simulink model "pipelined_simon"  (R2015b)
settings: Solver=FixedStepDiscrete  SolverMode=SingleTasking  StartTime=0.0  StopTime=5e-4  RelTol=1e-3
undefined symbols (not defined in the file or in its folder): a, b
libraries: shlslibv1 x1320
(part 1 of 6)
settings Model: synDspstartup=OK  Creator=pgali  LastModifiedBy=vchand32
settings DataIOCC: SaveOutput=off  SignalLogging=off  SaveTime=off
settings OptimizationCC: DefaultParameterBehavior=Inlined
settings DebuggingCC: AlgebraicLoopMsg=error  InheritedTsInSrcMsg=none

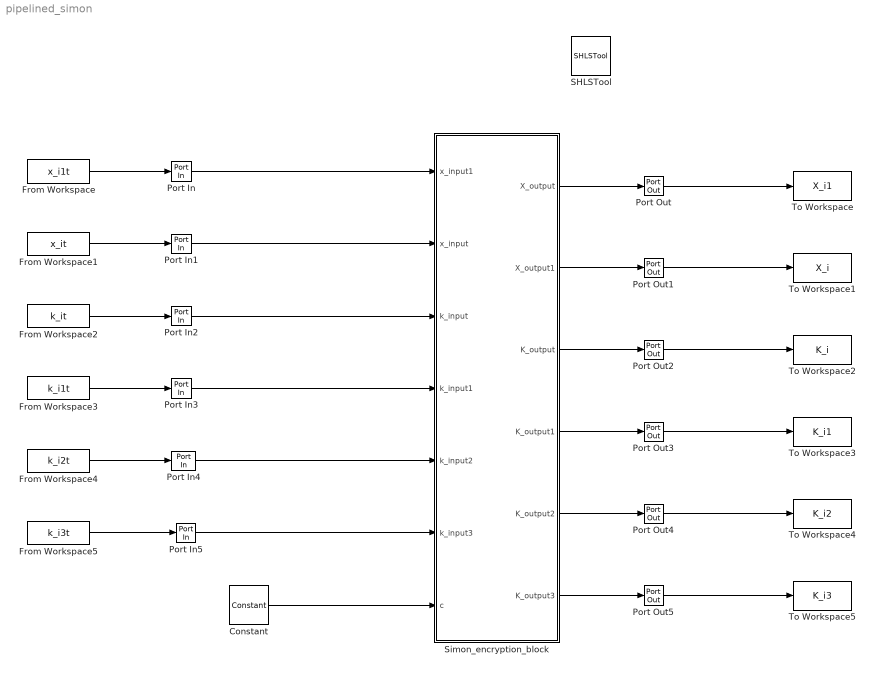
== system pipelined_simon ==
  Constant : shlslibv1/Sources/Constant  syn_cst_val=65532  syn_cst_format=Automatic  syn_cst_wl=1  syn_cst_fl=0  syn_cst_dt=unsigned  syn_cst_rnd=on  syn_cst_st=1/1040.5e6  synBlockType=primitive  synLatency=0  synBlockId=15
  From Workspace : FromWorkspace  VariableName=x_i1t  SampleTime=0
  From Workspace1 : FromWorkspace  VariableName=x_it  SampleTime=0
  From Workspace2 : FromWorkspace  VariableName=k_it  SampleTime=0
  From Workspace3 : FromWorkspace  VariableName=k_i1t  SampleTime=0
  From Workspace4 : FromWorkspace  VariableName=k_i2t  SampleTime=0
  From Workspace5 : FromWorkspace  VariableName=k_i3t  SampleTime=0
  Port In{,1..5} (6 alike) : shlslibv1/Ports & Subsystems/Port In  syn_out_wl=16  syn_out_fl=0  syn_out_dt=unsigned  syn_out_st=1/1040.5e6  syn_capture=on  syn_register=on  syn_out_sat=off  syn_out_rnd=on  synBlockType=port  synLatency=1  synBlockId=0
  Port Out{,1..5} (6 alike) : shlslibv1/Ports & Subsystems/Port Out  syn_capture=on  syn_register=on  synBlockType=port  synLatency=1  synBlockId=1
  SHLSTool : shlslibv1/SHLSTool  synBlockType=tool  syn_dsp_mode=FPGA
  "Simon_encryption_block " : Subsystem
  To Workspace : ToWorkspace  VariableName=X_i1  SaveFormat=Structure With Time  SampleTime=-1
  To Workspace1 : ToWorkspace  VariableName=X_i  SaveFormat=Structure With Time  SampleTime=-1
  To Workspace2 : ToWorkspace  VariableName=K_i  SaveFormat=Structure With Time  SampleTime=-1
  To Workspace3 : ToWorkspace  VariableName=K_i1  SaveFormat=Structure With Time  SampleTime=-1
  To Workspace4 : ToWorkspace  VariableName=K_i2  SaveFormat=Structure With Time  SampleTime=-1
  To Workspace5 : ToWorkspace  VariableName=K_i3  SaveFormat=Structure With Time  SampleTime=-1
  wires:
  From Workspace1/1 -> Port In1/1
  From Workspace2/1 -> Port In2/1
  From Workspace/1 -> Port In/1
  From Workspace3/1 -> Port In3/1
  From Workspace4/1 -> Port In4/1
  From Workspace5/1 -> Port In5/1
  Port In/1 -> "Simon_encryption_block "/1(x_input1)
  Port In1/1 -> "Simon_encryption_block "/2(x_input)
  Port In2/1 -> "Simon_encryption_block "/3(k_input)
  Port In3/1 -> "Simon_encryption_block "/4(k_input1)
  Port In4/1 -> "Simon_encryption_block "/5(k_input2)
  Port In5/1 -> "Simon_encryption_block "/6(k_input3)
  Port Out/1 -> To Workspace/1
  Port Out1/1 -> To Workspace1/1
  Port Out3/1 -> To Workspace3/1
  Port Out4/1 -> To Workspace4/1
  Port Out5/1 -> To Workspace5/1
  Port Out2/1 -> To Workspace2/1
  "Simon_encryption_block "/1(X_output) -> Port Out/1
  "Simon_encryption_block "/2(X_output1) -> Port Out1/1
  "Simon_encryption_block "/3(K_output) -> Port Out2/1
  "Simon_encryption_block "/4(K_output1) -> Port Out3/1
  "Simon_encryption_block "/5(K_output2) -> Port Out4/1
  "Simon_encryption_block "/6(K_output3) -> Port Out5/1
  Constant/1 -> "Simon_encryption_block "/7(c)

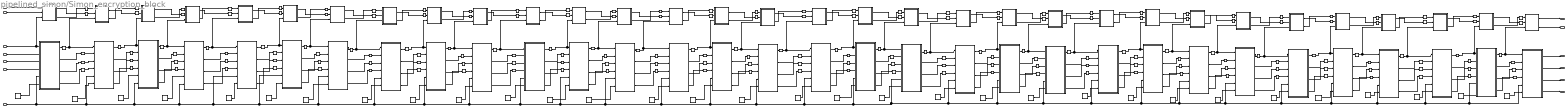
== system pipelined_simon/Simon_encryption_block  ==
  x_input1 : Inport
  x_input : Inport  Port=2
  k_input : Inport  Port=3
  k_input1 : Inport  Port=4
  k_input2 : Inport  Port=5
  k_input3 : Inport  Port=6
  c : Inport  Port=7
  Delay{1..186} (186 alike) : shlslibv1/Memories/Delay  syn_delay_val=1  synBlockType=primitive  synLatency=1  synBlockId=104
  Key_expansion_block : Subsystem
  Key_expansion_block1 : Subsystem
  Key_expansion_block10 : Subsystem
  Key_expansion_block11 : Subsystem
  Key_expansion_block12 : Subsystem
  Key_expansion_block13 : Subsystem
  Key_expansion_block14 : Subsystem
  Key_expansion_block15 : Subsystem
  Key_expansion_block16 : Subsystem
  Key_expansion_block17 : Subsystem
  Key_expansion_block18 : Subsystem
  Key_expansion_block19 : Subsystem
  Key_expansion_block2 : Subsystem
  Key_expansion_block20 : Subsystem
  Key_expansion_block21 : Subsystem
  Key_expansion_block22 : Subsystem
  Key_expansion_block23 : Subsystem
  Key_expansion_block24 : Subsystem
  Key_expansion_block25 : Subsystem
  Key_expansion_block26 : Subsystem
  Key_expansion_block27 : Subsystem
  Key_expansion_block28 : Subsystem
  Key_expansion_block29 : Subsystem
  Key_expansion_block3 : Subsystem
  Key_expansion_block30 : Subsystem
  Key_expansion_block31 : Subsystem
  Key_expansion_block4 : Subsystem
  Key_expansion_block5 : Subsystem
  Key_expansion_block6 : Subsystem
  Key_expansion_block7 : Subsystem
  Key_expansion_block8 : Subsystem
  Key_expansion_block9 : Subsystem
  Round_block : Subsystem
  Round_block1 : Subsystem
  Round_block10 : Subsystem
  Round_block11 : Subsystem
  Round_block12 : Subsystem
  Round_block13 : Subsystem
  Round_block14 : Subsystem
  Round_block15 : Subsystem
  Round_block16 : Subsystem
  Round_block17 : Subsystem
  Round_block18 : Subsystem
  Round_block19 : Subsystem
  Round_block2 : Subsystem
  Round_block20 : Subsystem
  Round_block21 : Subsystem
  Round_block22 : Subsystem
  Round_block23 : Subsystem
  Round_block24 : Subsystem
  Round_block25 : Subsystem
  Round_block26 : Subsystem
  Round_block27 : Subsystem
  Round_block28 : Subsystem
  Round_block29 : Subsystem
  Round_block3 : Subsystem
  Round_block30 : Subsystem
  Round_block31 : Subsystem
  Round_block4 : Subsystem
  Round_block5 : Subsystem
  Round_block6 : Subsystem
  Round_block7 : Subsystem
  Round_block8 : Subsystem
  Round_block9 : Subsystem
  Sequence{,1..4,6,10,13,15,17..18,23..25,28..29} (16 alike) : shlslibv1/Sources/Sequence  syn_seq_vec=[1]  syn_seq_wl=16  syn_seq_fl=0  syn_seq_dt=unsigned  syn_rst_port=off  syn_en_port=off  syn_seq_st=-1  synBlockType=custom  synLatency=1
  Sequence{5,7..9,11..12,14,16,19..22,26..27,30..31} (16 alike) : shlslibv1/Sources/Sequence  syn_seq_vec=[0]  syn_seq_wl=16  syn_seq_fl=0  syn_seq_dt=unsigned  syn_rst_port=off  syn_en_port=off  syn_seq_st=-1  synBlockType=custom  synLatency=1
  X_output : Outport
  X_output1 : Outport  Port=2
  K_output : Outport  Port=3
  K_output1 : Outport  Port=4
  K_output2 : Outport  Port=5
  K_output3 : Outport  Port=6
  wires:
  Key_expansion_block/2(Key_output1) -> Delay11/1
  Key_expansion_block/3(Key_output2) -> Delay12/1
  Key_expansion_block/4(Key_output3) -> Delay13/1
  x_input1/1 -> Round_block/1(" x_input1")
  x_input/1 -> Round_block/2(x_input)
  k_input/1 -> Round_block/3(k_i), Key_expansion_block/1(key_input)
  k_input1/1 -> Key_expansion_block/2(key_input1)
  k_input2/1 -> Key_expansion_block/3(key_input2)
  k_input3/1 -> Key_expansion_block/4(key_input3)
  Round_block/2(X_output) -> Delay7/1
  Round_block/1(X_output1) -> Delay8/1
  Round_block1/1(X_output1) -> Delay15/1
  Round_block1/2(X_output) -> Delay14/1
  Key_expansion_block1/2(Key_output1) -> Delay18/1
  Key_expansion_block1/3(Key_output2) -> Delay19/1
  Key_expansion_block1/4(Key_output3) -> Delay20/1
  Round_block2/1(X_output1) -> Delay22/1
  Round_block2/2(X_output) -> Delay21/1
  Key_expansion_block2/2(Key_output1) -> Delay25/1
  Key_expansion_block2/3(Key_output2) -> Delay26/1
  Key_expansion_block2/4(Key_output3) -> Delay27/1
  Delay7/1 -> Round_block1/1(" x_input1")
  Delay8/1 -> Round_block1/2(x_input)
  Key_expansion_block/1(Key_output) -> Delay9/1
  Delay11/1 -> Key_expansion_block1/2(key_input1)
  Delay12/1 -> Key_expansion_block1/3(key_input2)
  Delay13/1 -> Key_expansion_block1/4(key_input3)
  Delay14/1 -> Round_block2/1(" x_input1")
  Delay15/1 -> Round_block2/2(x_input)
  Key_expansion_block1/1(Key_output) -> Delay10/1
  Delay18/1 -> Key_expansion_block2/2(key_input1)
  Delay19/1 -> Key_expansion_block2/3(key_input2)
  Delay20/1 -> Key_expansion_block2/4(key_input3)
  Delay21/1 -> Round_block3/1(" x_input1")
  Delay22/1 -> Round_block3/2(x_input)
  Key_expansion_block2/1(Key_output) -> Delay16/1
  Delay25/1 -> Key_expansion_block3/2(key_input1)
  Delay26/1 -> Key_expansion_block3/3(key_input2)
  Delay27/1 -> Key_expansion_block3/4(key_input3)
  Delay9/1 -> Round_block1/3(k_i), Key_expansion_block1/1(key_input)
  Delay10/1 -> Round_block2/3(k_i), Key_expansion_block2/1(key_input)
  Delay16/1 -> Round_block3/3(k_i), Key_expansion_block3/1(key_input)
  Key_expansion_block3/2(Key_output1) -> Delay2/1
  Key_expansion_block3/3(Key_output2) -> Delay3/1
  Key_expansion_block3/4(Key_output3) -> Delay4/1
  Round_block3/2(X_output) -> Delay34/1
  Round_block3/1(X_output1) -> Delay35/1
  Round_block4/1(X_output1) -> Delay6/1
  Round_block4/2(X_output) -> Delay5/1
  Key_expansion_block4/2(Key_output1) -> Delay23/1
  Key_expansion_block4/3(Key_output2) -> Delay24/1
  Key_expansion_block4/4(Key_output3) -> Delay28/1
  Round_block5/1(X_output1) -> Delay30/1
  Round_block5/2(X_output) -> Delay29/1
  Key_expansion_block5/2(Key_output1) -> Delay31/1
  Key_expansion_block5/3(Key_output2) -> Delay32/1
  Key_expansion_block5/4(Key_output3) -> Delay33/1
  Delay34/1 -> Round_block4/1(" x_input1")
  Delay35/1 -> Round_block4/2(x_input)
  Key_expansion_block3/1(Key_output) -> Delay36/1
  Delay2/1 -> Key_expansion_block4/2(key_input1)
  Delay3/1 -> Key_expansion_block4/3(key_input2)
  Delay4/1 -> Key_expansion_block4/4(key_input3)
  Delay5/1 -> Round_block5/1(" x_input1")
  Delay6/1 -> Round_block5/2(x_input)
  Key_expansion_block4/1(Key_output) -> Delay1/1
  Delay23/1 -> Key_expansion_block5/2(key_input1)
  Delay24/1 -> Key_expansion_block5/3(key_input2)
  Delay28/1 -> Key_expansion_block5/4(key_input3)
  Delay29/1 -> Round_block6/1(" x_input1")
  Delay30/1 -> Round_block6/2(x_input)
  Key_expansion_block5/1(Key_output) -> Delay17/1
  Delay31/1 -> Key_expansion_block6/2(key_input1)
  Delay32/1 -> Key_expansion_block6/3(key_input2)
  Delay33/1 -> Key_expansion_block6/4(key_input3)
  Delay36/1 -> Round_block4/3(k_i), Key_expansion_block4/1(key_input)
  Delay1/1 -> Round_block5/3(k_i), Key_expansion_block5/1(key_input)
  Delay17/1 -> Round_block6/3(k_i), Key_expansion_block6/1(key_input)
  Key_expansion_block6/2(Key_output1) -> Delay39/1
  Key_expansion_block6/3(Key_output2) -> Delay40/1
  Key_expansion_block6/4(Key_output3) -> Delay41/1
  Round_block6/2(X_output) -> Delay70/1
  Round_block6/1(X_output1) -> Delay71/1
  Round_block7/1(X_output1) -> Delay43/1
  Round_block7/2(X_output) -> Delay42/1
  Key_expansion_block7/2(Key_output1) -> Delay46/1
  Key_expansion_block7/3(Key_output2) -> Delay47/1
  Key_expansion_block7/4(Key_output3) -> Delay49/1
  Round_block8/1(X_output1) -> Delay51/1
  Round_block8/2(X_output) -> Delay50/1
  Key_expansion_block8/2(Key_output1) -> Delay54/1
  Key_expansion_block8/3(Key_output2) -> Delay55/1
  Key_expansion_block8/4(Key_output3) -> Delay56/1
  Delay70/1 -> Round_block7/1(" x_input1")
  Delay71/1 -> Round_block7/2(x_input)
  Key_expansion_block6/1(Key_output) -> Delay72/1
  Delay39/1 -> Key_expansion_block7/2(key_input1)
  Delay40/1 -> Key_expansion_block7/3(key_input2)
  Delay41/1 -> Key_expansion_block7/4(key_input3)
  Delay42/1 -> Round_block8/1(" x_input1")
  Delay43/1 -> Round_block8/2(x_input)
  Key_expansion_block7/1(Key_output) -> Delay38/1
  Delay46/1 -> Key_expansion_block8/2(key_input1)
  Delay47/1 -> Key_expansion_block8/3(key_input2)
  Delay49/1 -> Key_expansion_block8/4(key_input3)
  Delay50/1 -> Round_block9/1(" x_input1")
  Delay51/1 -> Round_block9/2(x_input)
  Key_expansion_block8/1(Key_output) -> Delay44/1
  Delay54/1 -> Key_expansion_block9/2(key_input1)
  Delay55/1 -> Key_expansion_block9/3(key_input2)
  Delay56/1 -> Key_expansion_block9/4(key_input3)
  Delay72/1 -> Round_block7/3(k_i), Key_expansion_block7/1(key_input)
  Delay38/1 -> Round_block8/3(k_i), Key_expansion_block8/1(key_input)
  Delay44/1 -> Round_block9/3(k_i), Key_expansion_block9/1(key_input)
  Key_expansion_block9/2(Key_output1) -> Delay48/1
  Key_expansion_block9/3(Key_output2) -> Delay59/1
  Key_expansion_block9/4(Key_output3) -> Delay67/1
  Round_block9/2(X_output) -> Delay64/1
  Round_block9/1(X_output1) -> Delay65/1
  Round_block10/1(X_output1) -> Delay69/1
  Round_block10/2(X_output) -> Delay68/1
  Key_expansion_block10/2(Key_output1) -> Delay52/1
  Key_expansion_block10/3(Key_output2) -> Delay53/1
  Key_expansion_block10/4(Key_output3) -> Delay57/1
  Round_block11/1(X_output1) -> Delay60/1
  Round_block11/2(X_output) -> Delay58/1
  Key_expansion_block11/2(Key_output1) -> Delay61/1
  Key_expansion_block11/3(Key_output2) -> Delay62/1
  Key_expansion_block11/4(Key_output3) -> Delay63/1
  Delay64/1 -> Round_block10/1(" x_input1")
  Delay65/1 -> Round_block10/2(x_input)
  Key_expansion_block9/1(Key_output) -> Delay66/1
  Delay48/1 -> Key_expansion_block10/2(key_input1)
  Delay59/1 -> Key_expansion_block10/3(key_input2)
  Delay67/1 -> Key_expansion_block10/4(key_input3)
  Delay68/1 -> Round_block11/1(" x_input1")
  Delay69/1 -> Round_block11/2(x_input)
  Key_expansion_block10/1(Key_output) -> Delay37/1
  Delay52/1 -> Key_expansion_block11/2(key_input1)
  Delay53/1 -> Key_expansion_block11/3(key_input2)
  Delay57/1 -> Key_expansion_block11/4(key_input3)
  Delay58/1 -> Round_block12/1(" x_input1")
  Delay60/1 -> Round_block12/2(x_input)
  Key_expansion_block11/1(Key_output) -> Delay45/1
  Delay61/1 -> Key_expansion_block12/2(key_input1)
  Delay62/1 -> Key_expansion_block12/3(key_input2)
  Delay63/1 -> Key_expansion_block12/4(key_input3)
  Delay66/1 -> Round_block10/3(k_i), Key_expansion_block10/1(key_input)
  Delay37/1 -> Round_block11/3(k_i), Key_expansion_block11/1(key_input)
  Delay45/1 -> Round_block12/3(k_i), Key_expansion_block12/1(key_input)
  Key_expansion_block12/2(Key_output1) -> Delay75/1
  Key_expansion_block12/3(Key_output2) -> Delay76/1
  Key_expansion_block12/4(Key_output3) -> Delay77/1
  Round_block12/2(X_output) -> Delay139/1
  Round_block12/1(X_output1) -> Delay143/1
  Round_block13/1(X_output1) -> Delay79/1
  Round_block13/2(X_output) -> Delay78/1
  Key_expansion_block13/2(Key_output1) -> Delay82/1
  Key_expansion_block13/3(Key_output2) -> Delay83/1
  Key_expansion_block13/4(Key_output3) -> Delay85/1
  Round_block14/1(X_output1) -> Delay87/1
  Round_block14/2(X_output) -> Delay86/1
  Key_expansion_block14/2(Key_output1) -> Delay90/1
  Key_expansion_block14/3(Key_output2) -> Delay91/1
  Key_expansion_block14/4(Key_output3) -> Delay92/1
  Delay139/1 -> Round_block13/1(" x_input1")
  Delay143/1 -> Round_block13/2(x_input)
  Key_expansion_block12/1(Key_output) -> Delay144/1
  Delay75/1 -> Key_expansion_block13/2(key_input1)
  Delay76/1 -> Key_expansion_block13/3(key_input2)
  Delay77/1 -> Key_expansion_block13/4(key_input3)
  Delay78/1 -> Round_block14/1(" x_input1")
  Delay79/1 -> Round_block14/2(x_input)
  Key_expansion_block13/1(Key_output) -> Delay74/1
  Delay82/1 -> Key_expansion_block14/2(key_input1)
  Delay83/1 -> Key_expansion_block14/3(key_input2)
  Delay85/1 -> Key_expansion_block14/4(key_input3)
  Delay86/1 -> Round_block15/1(" x_input1")
  Delay87/1 -> Round_block15/2(x_input)
  Key_expansion_block14/1(Key_output) -> Delay80/1
  Delay90/1 -> Key_expansion_block15/2(key_input1)
  Delay91/1 -> Key_expansion_block15/3(key_input2)
  Delay92/1 -> Key_expansion_block15/4(key_input3)
  Delay144/1 -> Round_block13/3(k_i), Key_expansion_block13/1(key_input)
  Delay74/1 -> Round_block14/3(k_i), Key_expansion_block14/1(key_input)
  Delay80/1 -> Round_block15/3(k_i), Key_expansion_block15/1(key_input)
  Key_expansion_block15/2(Key_output1) -> Delay84/1
  Key_expansion_block15/3(Key_output2) -> Delay95/1
  Key_expansion_block15/4(Key_output3) -> Delay106/1
  Round_block15/2(X_output) -> Delay100/1
  Round_block15/1(X_output1) -> Delay101/1
  Round_block16/1(X_output1) -> Delay128/1
  Round_block16/2(X_output) -> Delay117/1
  Key_expansion_block16/2(Key_output1) -> Delay88/1
  Key_expansion_block16/3(Key_output2) -> Delay89/1
  Key_expansion_block16/4(Key_output3) -> Delay93/1
  Round_block17/1(X_output1) -> Delay96/1
  Round_block17/2(X_output) -> Delay94/1
  Key_expansion_block17/2(Key_output1) -> Delay97/1
  Key_expansion_block17/3(Key_output2) -> Delay98/1
  Key_expansion_block17/4(Key_output3) -> Delay99/1
  Delay100/1 -> Round_block16/1(" x_input1")
  Delay101/1 -> Round_block16/2(x_input)
  Key_expansion_block15/1(Key_output) -> Delay102/1
  Delay84/1 -> Key_expansion_block16/2(key_input1)
  Delay95/1 -> Key_expansion_block16/3(key_input2)
  Delay106/1 -> Key_expansion_block16/4(key_input3)
  Delay117/1 -> Round_block17/1(" x_input1")
  Delay128/1 -> Round_block17/2(x_input)
  Key_expansion_block16/1(Key_output) -> Delay73/1
  Delay88/1 -> Key_expansion_block17/2(key_input1)
  Delay89/1 -> Key_expansion_block17/3(key_input2)
  Delay93/1 -> Key_expansion_block17/4(key_input3)
  Delay94/1 -> Round_block18/1(" x_input1")
  Delay96/1 -> Round_block18/2(x_input)
  Key_expansion_block17/1(Key_output) -> Delay81/1
  Delay97/1 -> Key_expansion_block18/2(key_input1)
  Delay98/1 -> Key_expansion_block18/3(key_input2)
  Delay99/1 -> Key_expansion_block18/4(key_input3)
  Delay102/1 -> Round_block16/3(k_i), Key_expansion_block16/1(key_input)
  Delay73/1 -> Round_block17/3(k_i), Key_expansion_block17/1(key_input)
  Delay81/1 -> Round_block18/3(k_i), Key_expansion_block18/1(key_input)
  Key_expansion_block18/2(Key_output1) -> Delay105/1
  Key_expansion_block18/3(Key_output2) -> Delay107/1
  Key_expansion_block18/4(Key_output3) -> Delay108/1
  Round_block18/2(X_output) -> Delay140/1
  Round_block18/1(X_output1) -> Delay141/1
  Round_block19/1(X_output1) -> Delay110/1
  Round_block19/2(X_output) -> Delay109/1
  Key_expansion_block19/2(Key_output1) -> Delay113/1
  Key_expansion_block19/3(Key_output2) -> Delay114/1
  Key_expansion_block19/4(Key_output3) -> Delay116/1
  Round_block20/1(X_output1) -> Delay119/1
  Round_block20/2(X_output) -> Delay118/1
  Key_expansion_block20/2(Key_output1) -> Delay122/1
  Key_expansion_block20/3(Key_output2) -> Delay123/1
  Key_expansion_block20/4(Key_output3) -> Delay124/1
  Delay140/1 -> Round_block19/1(" x_input1")
  Delay141/1 -> Round_block19/2(x_input)
  Key_expansion_block18/1(Key_output) -> Delay142/1
  Delay105/1 -> Key_expansion_block19/2(key_input1)
  Delay107/1 -> Key_expansion_block19/3(key_input2)
  Delay108/1 -> Key_expansion_block19/4(key_input3)
  Delay109/1 -> Round_block20/1(" x_input1")
  Delay110/1 -> Round_block20/2(x_input)
  Key_expansion_block19/1(Key_output) -> Delay104/1
  Delay113/1 -> Key_expansion_block20/2(key_input1)
  Delay114/1 -> Key_expansion_block20/3(key_input2)
  Delay116/1 -> Key_expansion_block20/4(key_input3)
  Delay118/1 -> Round_block21/1(" x_input1")
  Delay119/1 -> Round_block21/2(x_input)
  Key_expansion_block20/1(Key_output) -> Delay111/1
  Delay122/1 -> Key_expansion_block21/2(key_input1)
  Delay123/1 -> Key_expansion_block21/3(key_input2)
  Delay124/1 -> Key_expansion_block21/4(key_input3)
  Delay142/1 -> Round_block19/3(k_i), Key_expansion_block19/1(key_input)
  Delay104/1 -> Round_block20/3(k_i), Key_expansion_block20/1(key_input)
  Delay111/1 -> Round_block21/3(k_i), Key_expansion_block21/1(key_input)
  Key_expansion_block21/2(Key_output1) -> Delay115/1
  Key_expansion_block21/3(Key_output2) -> Delay127/1
  Key_expansion_block21/4(Key_output3) -> Delay136/1
  Round_block21/2(X_output) -> Delay133/1
  Round_block21/1(X_output1) -> Delay134/1
  Round_block22/1(X_output1) -> Delay138/1
  Round_block22/2(X_output) -> Delay137/1
  Key_expansion_block22/2(Key_output1) -> Delay120/1
  Key_expansion_block22/3(Key_output2) -> Delay121/1
  Key_expansion_block22/4(Key_output3) -> Delay125/1
  Round_block23/1(X_output1) -> Delay129/1
  Round_block23/2(X_output) -> Delay126/1
  Key_expansion_block23/2(Key_output1) -> Delay130/1
  Key_expansion_block23/3(Key_output2) -> Delay131/1
  Key_expansion_block23/4(Key_output3) -> Delay132/1
  Delay133/1 -> Round_block22/1(" x_input1")
  Delay134/1 -> Round_block22/2(x_input)
  Key_expansion_block21/1(Key_output) -> Delay135/1
  Delay115/1 -> Key_expansion_block22/2(key_input1)
  Delay127/1 -> Key_expansion_block22/3(key_input2)
  Delay136/1 -> Key_expansion_block22/4(key_input3)
  Delay137/1 -> Round_block23/1(" x_input1")
  Delay138/1 -> Round_block23/2(x_input)
  Key_expansion_block22/1(Key_output) -> Delay103/1
  Delay120/1 -> Key_expansion_block23/2(key_input1)
  Delay121/1 -> Key_expansion_block23/3(key_input2)
  Delay125/1 -> Key_expansion_block23/4(key_input3)
  Delay126/1 -> Round_block24/1(" x_input1")
  Delay129/1 -> Round_block24/2(x_input)
  Key_expansion_block23/1(Key_output) -> Delay112/1
  Delay130/1 -> Key_expansion_block24/2(key_input1)
  Delay131/1 -> Key_expansion_block24/3(key_input2)
  Delay132/1 -> Key_expansion_block24/4(key_input3)
  Delay135/1 -> Round_block22/3(k_i), Key_expansion_block22/1(key_input)
  Delay103/1 -> Round_block23/3(k_i), Key_expansion_block23/1(key_input)
  Delay112/1 -> Round_block24/3(k_i), Key_expansion_block24/1(key_input)
  Round_block24/1(X_output1) -> Delay183/1
  Round_block24/2(X_output) -> Delay182/1
  Key_expansion_block24/2(Key_output1) -> Delay184/1
  Key_expansion_block24/3(Key_output2) -> Delay185/1
  Key_expansion_block24/4(Key_output3) -> Delay186/1
  Delay182/1 -> Round_block25/1(" x_input1")
  Delay183/1 -> Round_block25/2(x_input)
  Key_expansion_block24/1(Key_output) -> Delay181/1
  Delay184/1 -> Key_expansion_block25/2(key_input1)
  Delay185/1 -> Key_expansion_block25/3(key_input2)
  Delay186/1 -> Key_expansion_block25/4(key_input3)
  Delay181/1 -> Round_block25/3(k_i), Key_expansion_block25/1(key_input)
  Key_expansion_block25/2(Key_output1) -> Delay147/1
  Key_expansion_block25/3(Key_output2) -> Delay148/1
  Key_expansion_block25/4(Key_output3) -> Delay149/1
  Sequence27/1 -> Key_expansion_block27/6(z)
  Sequence28/1 -> Key_expansion_block28/6(z)
  Round_block25/2(X_output) -> Delay178/1
  Round_block25/1(X_output1) -> Delay179/1
  Round_block26/1(X_output1) -> Delay151/1
  Round_block26/2(X_output) -> Delay150/1
  Key_expansion_block26/2(Key_output1) -> Delay154/1
  Key_expansion_block26/3(Key_output2) -> Delay155/1
  Key_expansion_block26/4(Key_output3) -> Delay157/1
  Round_block27/1(X_output1) -> Delay159/1
  Round_block27/2(X_output) -> Delay158/1
  Key_expansion_block27/2(Key_output1) -> Delay162/1
  Key_expansion_block27/3(Key_output2) -> Delay163/1
  Key_expansion_block27/4(Key_output3) -> Delay164/1
  Delay178/1 -> Round_block26/1(" x_input1")
  Delay179/1 -> Round_block26/2(x_input)
  Key_expansion_block25/1(Key_output) -> Delay180/1
  Delay147/1 -> Key_expansion_block26/2(key_input1)
  Delay148/1 -> Key_expansion_block26/3(key_input2)
  Delay149/1 -> Key_expansion_block26/4(key_input3)
  Delay150/1 -> Round_block27/1(" x_input1")
  Delay151/1 -> Round_block27/2(x_input)
  Key_expansion_block26/1(Key_output) -> Delay146/1
  Delay154/1 -> Key_expansion_block27/2(key_input1)
  Delay155/1 -> Key_expansion_block27/3(key_input2)
  Delay157/1 -> Key_expansion_block27/4(key_input3)
  Delay158/1 -> Round_block28/1(" x_input1")
  Delay159/1 -> Round_block28/2(x_input)
  Key_expansion_block27/1(Key_output) -> Delay152/1
  Delay162/1 -> Key_expansion_block28/2(key_input1)
  Delay163/1 -> Key_expansion_block28/3(key_input2)
  Delay164/1 -> Key_expansion_block28/4(key_input3)
  Delay180/1 -> Round_block26/3(k_i), Key_expansion_block26/1(key_input)
  Delay146/1 -> Round_block27/3(k_i), Key_expansion_block27/1(key_input)
  Delay152/1 -> Round_block28/3(k_i), Key_expansion_block28/1(key_input)
  Key_expansion_block28/2(Key_output1) -> Delay156/1
  Key_expansion_block28/3(Key_output2) -> Delay167/1
  Key_expansion_block28/4(Key_output3) -> Delay175/1
  Sequence30/1 -> Key_expansion_block30/6(z)
  Round_block28/2(X_output) -> Delay172/1
  Round_block28/1(X_output1) -> Delay173/1
  Round_block29/1(X_output1) -> Delay177/1
  Round_block29/2(X_output) -> Delay176/1
  Key_expansion_block29/2(Key_output1) -> Delay160/1
  Key_expansion_block29/3(Key_output2) -> Delay161/1
  Key_expansion_block29/4(Key_output3) -> Delay165/1
  Round_block30/1(X_output1) -> Delay168/1
  Round_block30/2(X_output) -> Delay166/1
  Key_expansion_block30/2(Key_output1) -> Delay169/1
  Key_expansion_block30/3(Key_output2) -> Delay170/1
  Key_expansion_block30/4(Key_output3) -> Delay171/1
  Delay172/1 -> Round_block29/1(" x_input1")
  Delay173/1 -> Round_block29/2(x_input)
  Key_expansion_block28/1(Key_output) -> Delay174/1
  Delay156/1 -> Key_expansion_block29/2(key_input1)
  Delay167/1 -> Key_expansion_block29/3(key_input2)
  Delay175/1 -> Key_expansion_block29/4(key_input3)
  Delay176/1 -> Round_block30/1(" x_input1")
  Delay177/1 -> Round_block30/2(x_input)
  Key_expansion_block29/1(Key_output) -> Delay145/1
  Delay160/1 -> Key_expansion_block30/2(key_input1)
  Delay161/1 -> Key_expansion_block30/3(key_input2)
  Delay165/1 -> Key_expansion_block30/4(key_input3)
  Delay166/1 -> Round_block31/1(" x_input1")
  Delay168/1 -> Round_block31/2(x_input)
  Key_expansion_block30/1(Key_output) -> Delay153/1
  Delay169/1 -> Key_expansion_block31/2(key_input1)
  Delay170/1 -> Key_expansion_block31/3(key_input2)
  Delay171/1 -> Key_expansion_block31/4(key_input3)
  Delay174/1 -> Round_block29/3(k_i), Key_expansion_block29/1(key_input)
  Delay145/1 -> Round_block30/3(k_i), Key_expansion_block30/1(key_input)
  Delay153/1 -> Round_block31/3(k_i), Key_expansion_block31/1(key_input)
  c/1 -> Key_expansion_block1/5(c), Key_expansion_block2/6(z), Key_expansion_block3/6(z), Key_expansion_block4/5(c), Key_expansion_block5/5(c), Key_expansion_block6/5(c), Key_expansion_block7/5(c), Key_expansion_block8/5(c), Key_expansion_block9/5(c), Key_expansion_block10/5(c), Key_expansion_block11/5(c), Key_expansion_block12/5(c), Key_expansion_block13/5(c), Key_expansion_block14/5(c), Key_expansion_block15/5(c), Key_expansion_block16/5(c), Key_expansion_block17/5(c), Key_expansion_block18/5(c), Key_expansion_block19/5(c), Key_expansion_block20/5(c), Key_expansion_block21/5(c), Key_expansion_block22/5(c), Key_expansion_block23/5(c), Key_expansion_block24/5(c), Key_expansion_block25/5(c), Key_expansion_block26/5(c), Key_expansion_block27/5(c), Key_expansion_block28/5(c), Key_expansion_block29/5(c), Key_expansion_block30/5(c), Key_expansion_block31/5(c), Key_expansion_block/5(c)
  Sequence/1 -> Key_expansion_block/6(z)
  Sequence1/1 -> Key_expansion_block1/6(z)
  Sequence2/1 -> Key_expansion_block2/5(c)
  Sequence3/1 -> Key_expansion_block3/5(c)
  Sequence4/1 -> Key_expansion_block4/6(z)
  Sequence5/1 -> Key_expansion_block5/6(z)
  Sequence6/1 -> Key_expansion_block6/6(z)
  Sequence7/1 -> Key_expansion_block7/6(z)
  Sequence8/1 -> Key_expansion_block8/6(z)
  Sequence9/1 -> Key_expansion_block9/6(z)
  Sequence10/1 -> Key_expansion_block10/6(z)
  Sequence11/1 -> Key_expansion_block11/6(z)
  Sequence12/1 -> Key_expansion_block12/6(z)
  Sequence13/1 -> Key_expansion_block13/6(z)
  Sequence14/1 -> Key_expansion_block14/6(z)
  Sequence15/1 -> Key_expansion_block15/6(z)
  Sequence16/1 -> Key_expansion_block16/6(z)
  Sequence17/1 -> Key_expansion_block17/6(z)
  Sequence18/1 -> Key_expansion_block18/6(z)
  Sequence19/1 -> Key_expansion_block19/6(z)
  Sequence20/1 -> Key_expansion_block20/6(z)
  Sequence21/1 -> Key_expansion_block21/6(z)
  Sequence22/1 -> Key_expansion_block22/6(z)
  Sequence23/1 -> Key_expansion_block23/6(z)
  Sequence29/1 -> Key_expansion_block29/6(z)
  Sequence26/1 -> Key_expansion_block26/6(z)
  Sequence31/1 -> Key_expansion_block31/6(z)
  Sequence25/1 -> Key_expansion_block25/6(z)
  Sequence24/1 -> Key_expansion_block24/6(z)
  Round_block31/1(X_output1) -> X_output/1
  Round_block31/2(X_output) -> X_output1/1
  Key_expansion_block31/1(Key_output) -> K_output/1
  Key_expansion_block31/2(Key_output1) -> K_output1/1
  Key_expansion_block31/3(Key_output2) -> K_output2/1
  Key_expansion_block31/4(Key_output3) -> K_output3/1

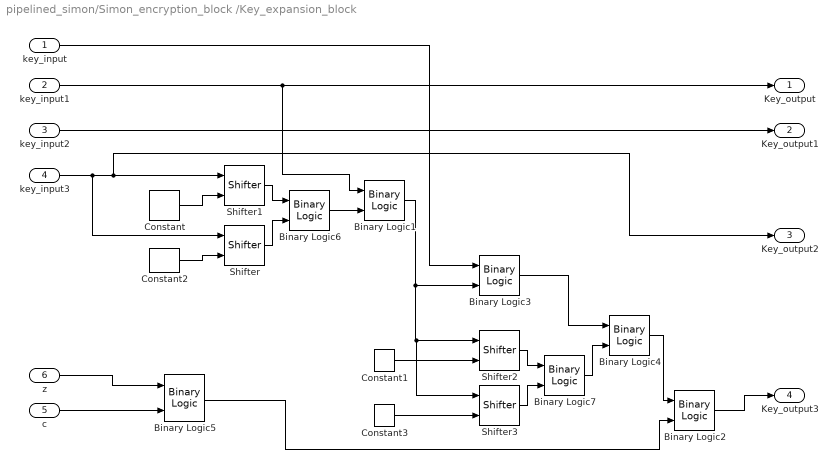
== system pipelined_simon/Simon_encryption_block /Key_expansion_block ==
  key_input : Inport
  key_input1 : Inport  Port=2
  key_input2 : Inport  Port=3
  key_input3 : Inport  Port=4
  c : Inport  Port=5
  z : Inport  Port=6
  Binary Logic{1..5} (5 alike) : shlslibv1/Math Functions/Binary Logic  syn_binlog_exp=a^b  synBlockType=primitive  synLatency=0  synBlockId=13
  Binary Logic6 : shlslibv1/Math Functions/Binary Logic  syn_binlog_exp=a|b  synBlockType=primitive  synLatency=0  synBlockId=13
  Binary Logic7 : shlslibv1/Math Functions/Binary Logic  syn_binlog_exp=a|b  synBlockType=primitive  synLatency=0  synBlockId=13
  Constant : shlslibv1/Sources/Constant  syn_cst_val=3  syn_cst_format=Specify  syn_cst_wl=4  syn_cst_fl=0  syn_cst_dt=unsigned  syn_cst_rnd=on  syn_cst_st=-1  synBlockType=primitive  synLatency=0  synBlockId=15
  Constant1 : shlslibv1/Sources/Constant  syn_cst_val=1  syn_cst_format=Specify  syn_cst_wl=4  syn_cst_fl=0  syn_cst_dt=unsigned  syn_cst_rnd=on  syn_cst_st=-1  synBlockType=primitive  synLatency=0  synBlockId=15
  Constant2 : shlslibv1/Sources/Constant  syn_cst_val=13  syn_cst_format=Specify  syn_cst_wl=4  syn_cst_fl=0  syn_cst_dt=unsigned  syn_cst_rnd=on  syn_cst_st=-1  synBlockType=primitive  synLatency=0  synBlockId=15
  Constant3 : shlslibv1/Sources/Constant  syn_cst_val=15  syn_cst_format=Specify  syn_cst_wl=4  syn_cst_fl=0  syn_cst_dt=unsigned  syn_cst_rnd=on  syn_cst_st=-1  synBlockType=primitive  synLatency=0  synBlockId=15
  Shifter : shlslibv1/Math Functions/Shifter  syn_shifter_opr=<<  syn_out_f=Automatic  syn_out_wl=16  syn_out_fl=8  syn_out_dt=signed  synBlockType=primitive  synLatency=0  synBlockId=12
  Shifter1 : shlslibv1/Math Functions/Shifter  syn_shifter_opr=>>  syn_out_f=Automatic  syn_out_wl=16  syn_out_fl=8  syn_out_dt=signed  synBlockType=primitive  synLatency=0  synBlockId=12
  Shifter2 : shlslibv1/Math Functions/Shifter  syn_shifter_opr=>>  syn_out_f=Automatic  syn_out_wl=16  syn_out_fl=8  syn_out_dt=signed  synBlockType=primitive  synLatency=0  synBlockId=12
  Shifter3 : shlslibv1/Math Functions/Shifter  syn_shifter_opr=<<  syn_out_f=Automatic  syn_out_wl=16  syn_out_fl=8  syn_out_dt=signed  synBlockType=primitive  synLatency=0  synBlockId=12
  Key_output : Outport
  Key_output1 : Outport  Port=2
  Key_output2 : Outport  Port=3
  Key_output3 : Outport  Port=4
  wires:
  Binary Logic1/1 -> Shifter3/1, Shifter2/1, Binary Logic3/2
  Constant/1 -> Shifter1/2
  Constant1/1 -> Shifter2/2
  Binary Logic2/1 -> Key_output3/1
  Binary Logic4/1 -> Binary Logic2/1
  key_input/1 -> Binary Logic3/1
  key_input1/1 -> Key_output/1, Binary Logic1/1
  z/1 -> Binary Logic5/1
  c/1 -> Binary Logic5/2
  key_input2/1 -> Key_output1/1
  key_input3/1 -> Shifter/1, Shifter1/1, Key_output2/1
  Binary Logic3/1 -> Binary Logic4/1
  Binary Logic5/1 -> Binary Logic2/2
  Constant2/1 -> Shifter/2
  Shifter1/1 -> Binary Logic6/1
  Shifter/1 -> Binary Logic6/2
  Binary Logic6/1 -> Binary Logic1/2
  Constant3/1 -> Shifter3/2
  Shifter2/1 -> Binary Logic7/1
  Shifter3/1 -> Binary Logic7/2
  Binary Logic7/1 -> Binary Logic4/2

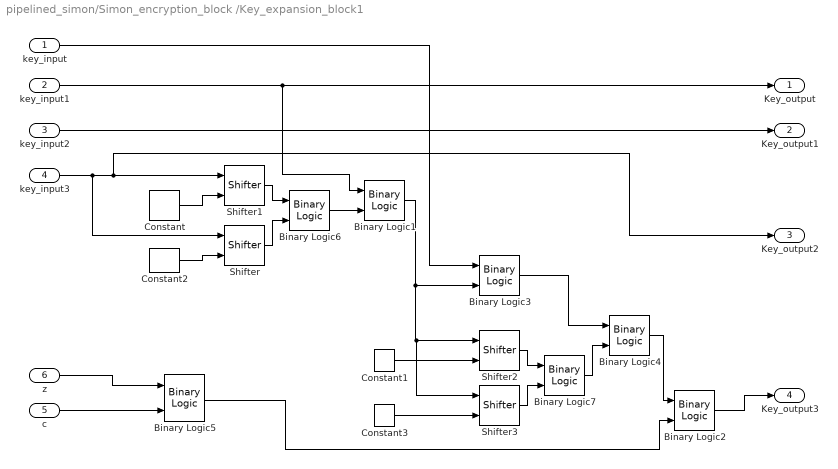
== system pipelined_simon/Simon_encryption_block /Key_expansion_block1 ==
  key_input : Inport
  key_input1 : Inport  Port=2
  key_input2 : Inport  Port=3
  key_input3 : Inport  Port=4
  c : Inport  Port=5
  z : Inport  Port=6
  Binary Logic{1..5} (5 alike) : shlslibv1/Math Functions/Binary Logic  syn_binlog_exp=a^b  synBlockType=primitive  synLatency=0  synBlockId=13
  Binary Logic6 : shlslibv1/Math Functions/Binary Logic  syn_binlog_exp=a|b  synBlockType=primitive  synLatency=0  synBlockId=13
  Binary Logic7 : shlslibv1/Math Functions/Binary Logic  syn_binlog_exp=a|b  synBlockType=primitive  synLatency=0  synBlockId=13
  Constant : shlslibv1/Sources/Constant  syn_cst_val=3  syn_cst_format=Specify  syn_cst_wl=4  syn_cst_fl=0  syn_cst_dt=unsigned  syn_cst_rnd=on  syn_cst_st=-1  synBlockType=primitive  synLatency=0  synBlockId=15
  Constant1 : shlslibv1/Sources/Constant  syn_cst_val=1  syn_cst_format=Specify  syn_cst_wl=4  syn_cst_fl=0  syn_cst_dt=unsigned  syn_cst_rnd=on  syn_cst_st=-1  synBlockType=primitive  synLatency=0  synBlockId=15
  Constant2 : shlslibv1/Sources/Constant  syn_cst_val=13  syn_cst_format=Specify  syn_cst_wl=4  syn_cst_fl=0  syn_cst_dt=unsigned  syn_cst_rnd=on  syn_cst_st=-1  synBlockType=primitive  synLatency=0  synBlockId=15
  Constant3 : shlslibv1/Sources/Constant  syn_cst_val=15  syn_cst_format=Specify  syn_cst_wl=4  syn_cst_fl=0  syn_cst_dt=unsigned  syn_cst_rnd=on  syn_cst_st=-1  synBlockType=primitive  synLatency=0  synBlockId=15
  Shifter : shlslibv1/Math Functions/Shifter  syn_shifter_opr=<<  syn_out_f=Automatic  syn_out_wl=16  syn_out_fl=8  syn_out_dt=signed  synBlockType=primitive  synLatency=0  synBlockId=12
  Shifter1 : shlslibv1/Math Functions/Shifter  syn_shifter_opr=>>  syn_out_f=Automatic  syn_out_wl=16  syn_out_fl=8  syn_out_dt=signed  synBlockType=primitive  synLatency=0  synBlockId=12
  Shifter2 : shlslibv1/Math Functions/Shifter  syn_shifter_opr=>>  syn_out_f=Automatic  syn_out_wl=16  syn_out_fl=8  syn_out_dt=signed  synBlockType=primitive  synLatency=0  synBlockId=12
  Shifter3 : shlslibv1/Math Functions/Shifter  syn_shifter_opr=<<  syn_out_f=Automatic  syn_out_wl=16  syn_out_fl=8  syn_out_dt=signed  synBlockType=primitive  synLatency=0  synBlockId=12
  Key_output : Outport
  Key_output1 : Outport  Port=2
  Key_output2 : Outport  Port=3
  Key_output3 : Outport  Port=4
  wires:
  Binary Logic1/1 -> Shifter3/1, Shifter2/1, Binary Logic3/2
  Constant/1 -> Shifter1/2
  Constant1/1 -> Shifter2/2
  Binary Logic2/1 -> Key_output3/1
  Binary Logic4/1 -> Binary Logic2/1
  key_input/1 -> Binary Logic3/1
  key_input1/1 -> Key_output/1, Binary Logic1/1
  z/1 -> Binary Logic5/1
  c/1 -> Binary Logic5/2
  key_input2/1 -> Key_output1/1
  key_input3/1 -> Shifter/1, Shifter1/1, Key_output2/1
  Binary Logic3/1 -> Binary Logic4/1
  Binary Logic5/1 -> Binary Logic2/2
  Constant2/1 -> Shifter/2
  Shifter1/1 -> Binary Logic6/1
  Shifter/1 -> Binary Logic6/2
  Binary Logic6/1 -> Binary Logic1/2
  Constant3/1 -> Shifter3/2
  Shifter2/1 -> Binary Logic7/1
  Shifter3/1 -> Binary Logic7/2
  Binary Logic7/1 -> Binary Logic4/2

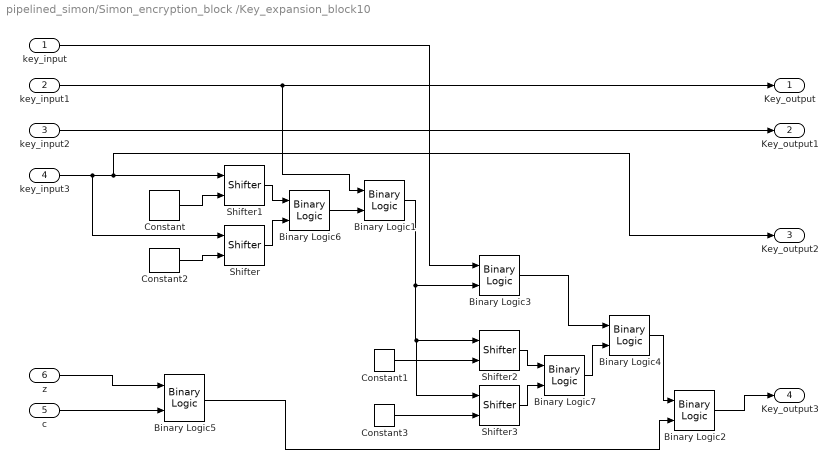
== system pipelined_simon/Simon_encryption_block /Key_expansion_block10 ==
  key_input : Inport
  key_input1 : Inport  Port=2
  key_input2 : Inport  Port=3
  key_input3 : Inport  Port=4
  c : Inport  Port=5
  z : Inport  Port=6
  Binary Logic{1..5} (5 alike) : shlslibv1/Math Functions/Binary Logic  syn_binlog_exp=a^b  synBlockType=primitive  synLatency=0  synBlockId=13
  Binary Logic6 : shlslibv1/Math Functions/Binary Logic  syn_binlog_exp=a|b  synBlockType=primitive  synLatency=0  synBlockId=13
  Binary Logic7 : shlslibv1/Math Functions/Binary Logic  syn_binlog_exp=a|b  synBlockType=primitive  synLatency=0  synBlockId=13
  Constant : shlslibv1/Sources/Constant  syn_cst_val=3  syn_cst_format=Specify  syn_cst_wl=4  syn_cst_fl=0  syn_cst_dt=unsigned  syn_cst_rnd=on  syn_cst_st=-1  synBlockType=primitive  synLatency=0  synBlockId=15
  Constant1 : shlslibv1/Sources/Constant  syn_cst_val=1  syn_cst_format=Specify  syn_cst_wl=4  syn_cst_fl=0  syn_cst_dt=unsigned  syn_cst_rnd=on  syn_cst_st=-1  synBlockType=primitive  synLatency=0  synBlockId=15
  Constant2 : shlslibv1/Sources/Constant  syn_cst_val=13  syn_cst_format=Specify  syn_cst_wl=4  syn_cst_fl=0  syn_cst_dt=unsigned  syn_cst_rnd=on  syn_cst_st=-1  synBlockType=primitive  synLatency=0  synBlockId=15
  Constant3 : shlslibv1/Sources/Constant  syn_cst_val=15  syn_cst_format=Specify  syn_cst_wl=4  syn_cst_fl=0  syn_cst_dt=unsigned  syn_cst_rnd=on  syn_cst_st=-1  synBlockType=primitive  synLatency=0  synBlockId=15
  Shifter : shlslibv1/Math Functions/Shifter  syn_shifter_opr=<<  syn_out_f=Automatic  syn_out_wl=16  syn_out_fl=8  syn_out_dt=signed  synBlockType=primitive  synLatency=0  synBlockId=12
  Shifter1 : shlslibv1/Math Functions/Shifter  syn_shifter_opr=>>  syn_out_f=Automatic  syn_out_wl=16  syn_out_fl=8  syn_out_dt=signed  synBlockType=primitive  synLatency=0  synBlockId=12
  Shifter2 : shlslibv1/Math Functions/Shifter  syn_shifter_opr=>>  syn_out_f=Automatic  syn_out_wl=16  syn_out_fl=8  syn_out_dt=signed  synBlockType=primitive  synLatency=0  synBlockId=12
  Shifter3 : shlslibv1/Math Functions/Shifter  syn_shifter_opr=<<  syn_out_f=Automatic  syn_out_wl=16  syn_out_fl=8  syn_out_dt=signed  synBlockType=primitive  synLatency=0  synBlockId=12
  Key_output : Outport
  Key_output1 : Outport  Port=2
  Key_output2 : Outport  Port=3
  Key_output3 : Outport  Port=4
  wires:
  Binary Logic1/1 -> Shifter3/1, Shifter2/1, Binary Logic3/2
  Constant/1 -> Shifter1/2
  Constant1/1 -> Shifter2/2
  Binary Logic2/1 -> Key_output3/1
  Binary Logic4/1 -> Binary Logic2/1
  key_input/1 -> Binary Logic3/1
  key_input1/1 -> Key_output/1, Binary Logic1/1
  z/1 -> Binary Logic5/1
  c/1 -> Binary Logic5/2
  key_input2/1 -> Key_output1/1
  key_input3/1 -> Shifter/1, Shifter1/1, Key_output2/1
  Binary Logic3/1 -> Binary Logic4/1
  Binary Logic5/1 -> Binary Logic2/2
  Constant2/1 -> Shifter/2
  Shifter1/1 -> Binary Logic6/1
  Shifter/1 -> Binary Logic6/2
  Binary Logic6/1 -> Binary Logic1/2
  Constant3/1 -> Shifter3/2
  Shifter2/1 -> Binary Logic7/1
  Shifter3/1 -> Binary Logic7/2
  Binary Logic7/1 -> Binary Logic4/2

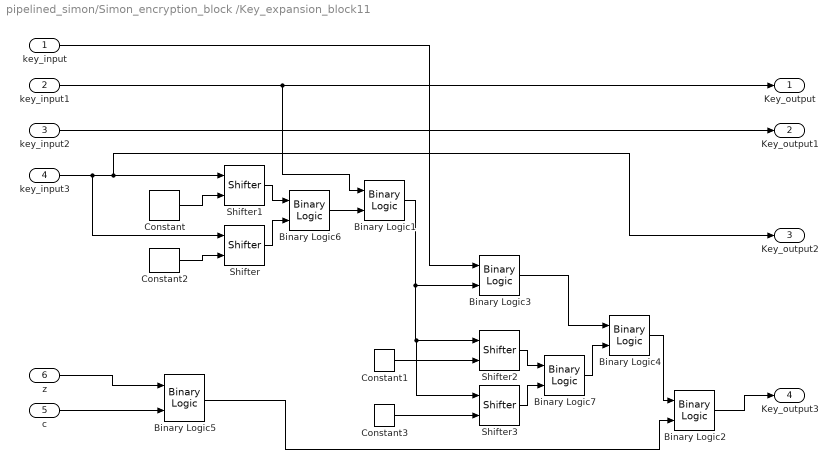
== system pipelined_simon/Simon_encryption_block /Key_expansion_block11 ==
  key_input : Inport
  key_input1 : Inport  Port=2
  key_input2 : Inport  Port=3
  key_input3 : Inport  Port=4
  c : Inport  Port=5
  z : Inport  Port=6
  Binary Logic{1..5} (5 alike) : shlslibv1/Math Functions/Binary Logic  syn_binlog_exp=a^b  synBlockType=primitive  synLatency=0  synBlockId=13
  Binary Logic6 : shlslibv1/Math Functions/Binary Logic  syn_binlog_exp=a|b  synBlockType=primitive  synLatency=0  synBlockId=13
  Binary Logic7 : shlslibv1/Math Functions/Binary Logic  syn_binlog_exp=a|b  synBlockType=primitive  synLatency=0  synBlockId=13
  Constant : shlslibv1/Sources/Constant  syn_cst_val=3  syn_cst_format=Specify  syn_cst_wl=4  syn_cst_fl=0  syn_cst_dt=unsigned  syn_cst_rnd=on  syn_cst_st=-1  synBlockType=primitive  synLatency=0  synBlockId=15
  Constant1 : shlslibv1/Sources/Constant  syn_cst_val=1  syn_cst_format=Specify  syn_cst_wl=4  syn_cst_fl=0  syn_cst_dt=unsigned  syn_cst_rnd=on  syn_cst_st=-1  synBlockType=primitive  synLatency=0  synBlockId=15
  Constant2 : shlslibv1/Sources/Constant  syn_cst_val=13  syn_cst_format=Specify  syn_cst_wl=4  syn_cst_fl=0  syn_cst_dt=unsigned  syn_cst_rnd=on  syn_cst_st=-1  synBlockType=primitive  synLatency=0  synBlockId=15
  Constant3 : shlslibv1/Sources/Constant  syn_cst_val=15  syn_cst_format=Specify  syn_cst_wl=4  syn_cst_fl=0  syn_cst_dt=unsigned  syn_cst_rnd=on  syn_cst_st=-1  synBlockType=primitive  synLatency=0  synBlockId=15
  Shifter : shlslibv1/Math Functions/Shifter  syn_shifter_opr=<<  syn_out_f=Automatic  syn_out_wl=16  syn_out_fl=8  syn_out_dt=signed  synBlockType=primitive  synLatency=0  synBlockId=12
  Shifter1 : shlslibv1/Math Functions/Shifter  syn_shifter_opr=>>  syn_out_f=Automatic  syn_out_wl=16  syn_out_fl=8  syn_out_dt=signed  synBlockType=primitive  synLatency=0  synBlockId=12
  Shifter2 : shlslibv1/Math Functions/Shifter  syn_shifter_opr=>>  syn_out_f=Automatic  syn_out_wl=16  syn_out_fl=8  syn_out_dt=signed  synBlockType=primitive  synLatency=0  synBlockId=12
  Shifter3 : shlslibv1/Math Functions/Shifter  syn_shifter_opr=<<  syn_out_f=Automatic  syn_out_wl=16  syn_out_fl=8  syn_out_dt=signed  synBlockType=primitive  synLatency=0  synBlockId=12
  Key_output : Outport
  Key_output1 : Outport  Port=2
  Key_output2 : Outport  Port=3
  Key_output3 : Outport  Port=4
  wires:
  Binary Logic1/1 -> Shifter3/1, Shifter2/1, Binary Logic3/2
  Constant/1 -> Shifter1/2
  Constant1/1 -> Shifter2/2
  Binary Logic2/1 -> Key_output3/1
  Binary Logic4/1 -> Binary Logic2/1
  key_input/1 -> Binary Logic3/1
  key_input1/1 -> Key_output/1, Binary Logic1/1
  z/1 -> Binary Logic5/1
  c/1 -> Binary Logic5/2
  key_input2/1 -> Key_output1/1
  key_input3/1 -> Shifter/1, Shifter1/1, Key_output2/1
  Binary Logic3/1 -> Binary Logic4/1
  Binary Logic5/1 -> Binary Logic2/2
  Constant2/1 -> Shifter/2
  Shifter1/1 -> Binary Logic6/1
  Shifter/1 -> Binary Logic6/2
  Binary Logic6/1 -> Binary Logic1/2
  Constant3/1 -> Shifter3/2
  Shifter2/1 -> Binary Logic7/1
  Shifter3/1 -> Binary Logic7/2
  Binary Logic7/1 -> Binary Logic4/2

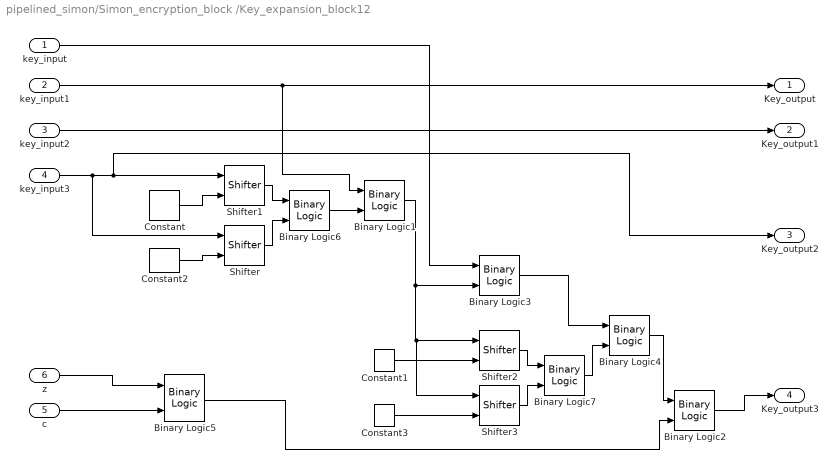
== system pipelined_simon/Simon_encryption_block /Key_expansion_block12 ==
  key_input : Inport
  key_input1 : Inport  Port=2
  key_input2 : Inport  Port=3
  key_input3 : Inport  Port=4
  c : Inport  Port=5
  z : Inport  Port=6
  Binary Logic{1..5} (5 alike) : shlslibv1/Math Functions/Binary Logic  syn_binlog_exp=a^b  synBlockType=primitive  synLatency=0  synBlockId=13
  Binary Logic6 : shlslibv1/Math Functions/Binary Logic  syn_binlog_exp=a|b  synBlockType=primitive  synLatency=0  synBlockId=13
  Binary Logic7 : shlslibv1/Math Functions/Binary Logic  syn_binlog_exp=a|b  synBlockType=primitive  synLatency=0  synBlockId=13
  Constant : shlslibv1/Sources/Constant  syn_cst_val=3  syn_cst_format=Specify  syn_cst_wl=4  syn_cst_fl=0  syn_cst_dt=unsigned  syn_cst_rnd=on  syn_cst_st=-1  synBlockType=primitive  synLatency=0  synBlockId=15
  Constant1 : shlslibv1/Sources/Constant  syn_cst_val=1  syn_cst_format=Specify  syn_cst_wl=4  syn_cst_fl=0  syn_cst_dt=unsigned  syn_cst_rnd=on  syn_cst_st=-1  synBlockType=primitive  synLatency=0  synBlockId=15
  Constant2 : shlslibv1/Sources/Constant  syn_cst_val=13  syn_cst_format=Specify  syn_cst_wl=4  syn_cst_fl=0  syn_cst_dt=unsigned  syn_cst_rnd=on  syn_cst_st=-1  synBlockType=primitive  synLatency=0  synBlockId=15
  Constant3 : shlslibv1/Sources/Constant  syn_cst_val=15  syn_cst_format=Specify  syn_cst_wl=4  syn_cst_fl=0  syn_cst_dt=unsigned  syn_cst_rnd=on  syn_cst_st=-1  synBlockType=primitive  synLatency=0  synBlockId=15
  Shifter : shlslibv1/Math Functions/Shifter  syn_shifter_opr=<<  syn_out_f=Automatic  syn_out_wl=16  syn_out_fl=8  syn_out_dt=signed  synBlockType=primitive  synLatency=0  synBlockId=12
  Shifter1 : shlslibv1/Math Functions/Shifter  syn_shifter_opr=>>  syn_out_f=Automatic  syn_out_wl=16  syn_out_fl=8  syn_out_dt=signed  synBlockType=primitive  synLatency=0  synBlockId=12
  Shifter2 : shlslibv1/Math Functions/Shifter  syn_shifter_opr=>>  syn_out_f=Automatic  syn_out_wl=16  syn_out_fl=8  syn_out_dt=signed  synBlockType=primitive  synLatency=0  synBlockId=12
  Shifter3 : shlslibv1/Math Functions/Shifter  syn_shifter_opr=<<  syn_out_f=Automatic  syn_out_wl=16  syn_out_fl=8  syn_out_dt=signed  synBlockType=primitive  synLatency=0  synBlockId=12
  Key_output : Outport
  Key_output1 : Outport  Port=2
  Key_output2 : Outport  Port=3
  Key_output3 : Outport  Port=4
  wires:
  Binary Logic1/1 -> Shifter3/1, Shifter2/1, Binary Logic3/2
  Constant/1 -> Shifter1/2
  Constant1/1 -> Shifter2/2
  Binary Logic2/1 -> Key_output3/1
  Binary Logic4/1 -> Binary Logic2/1
  key_input/1 -> Binary Logic3/1
  key_input1/1 -> Key_output/1, Binary Logic1/1
  z/1 -> Binary Logic5/1
  c/1 -> Binary Logic5/2
  key_input2/1 -> Key_output1/1
  key_input3/1 -> Shifter/1, Shifter1/1, Key_output2/1
  Binary Logic3/1 -> Binary Logic4/1
  Binary Logic5/1 -> Binary Logic2/2
  Constant2/1 -> Shifter/2
  Shifter1/1 -> Binary Logic6/1
  Shifter/1 -> Binary Logic6/2
  Binary Logic6/1 -> Binary Logic1/2
  Constant3/1 -> Shifter3/2
  Shifter2/1 -> Binary Logic7/1
  Shifter3/1 -> Binary Logic7/2
  Binary Logic7/1 -> Binary Logic4/2

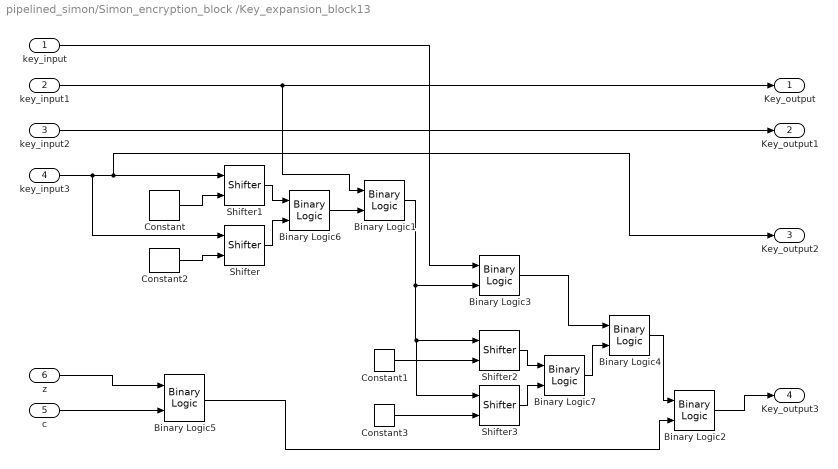
== system pipelined_simon/Simon_encryption_block /Key_expansion_block13 ==
  key_input : Inport
  key_input1 : Inport  Port=2
  key_input2 : Inport  Port=3
  key_input3 : Inport  Port=4
  c : Inport  Port=5
  z : Inport  Port=6
  Binary Logic{1..5} (5 alike) : shlslibv1/Math Functions/Binary Logic  syn_binlog_exp=a^b  synBlockType=primitive  synLatency=0  synBlockId=13
  Binary Logic6 : shlslibv1/Math Functions/Binary Logic  syn_binlog_exp=a|b  synBlockType=primitive  synLatency=0  synBlockId=13
  Binary Logic7 : shlslibv1/Math Functions/Binary Logic  syn_binlog_exp=a|b  synBlockType=primitive  synLatency=0  synBlockId=13
  Constant : shlslibv1/Sources/Constant  syn_cst_val=3  syn_cst_format=Specify  syn_cst_wl=4  syn_cst_fl=0  syn_cst_dt=unsigned  syn_cst_rnd=on  syn_cst_st=-1  synBlockType=primitive  synLatency=0  synBlockId=15
  Constant1 : shlslibv1/Sources/Constant  syn_cst_val=1  syn_cst_format=Specify  syn_cst_wl=4  syn_cst_fl=0  syn_cst_dt=unsigned  syn_cst_rnd=on  syn_cst_st=-1  synBlockType=primitive  synLatency=0  synBlockId=15
  Constant2 : shlslibv1/Sources/Constant  syn_cst_val=13  syn_cst_format=Specify  syn_cst_wl=4  syn_cst_fl=0  syn_cst_dt=unsigned  syn_cst_rnd=on  syn_cst_st=-1  synBlockType=primitive  synLatency=0  synBlockId=15
  Constant3 : shlslibv1/Sources/Constant  syn_cst_val=15  syn_cst_format=Specify  syn_cst_wl=4  syn_cst_fl=0  syn_cst_dt=unsigned  syn_cst_rnd=on  syn_cst_st=-1  synBlockType=primitive  synLatency=0  synBlockId=15
  Shifter : shlslibv1/Math Functions/Shifter  syn_shifter_opr=<<  syn_out_f=Automatic  syn_out_wl=16  syn_out_fl=8  syn_out_dt=signed  synBlockType=primitive  synLatency=0  synBlockId=12
  Shifter1 : shlslibv1/Math Functions/Shifter  syn_shifter_opr=>>  syn_out_f=Automatic  syn_out_wl=16  syn_out_fl=8  syn_out_dt=signed  synBlockType=primitive  synLatency=0  synBlockId=12
  Shifter2 : shlslibv1/Math Functions/Shifter  syn_shifter_opr=>>  syn_out_f=Automatic  syn_out_wl=16  syn_out_fl=8  syn_out_dt=signed  synBlockType=primitive  synLatency=0  synBlockId=12
  Shifter3 : shlslibv1/Math Functions/Shifter  syn_shifter_opr=<<  syn_out_f=Automatic  syn_out_wl=16  syn_out_fl=8  syn_out_dt=signed  synBlockType=primitive  synLatency=0  synBlockId=12
  Key_output : Outport
  Key_output1 : Outport  Port=2
  Key_output2 : Outport  Port=3
  Key_output3 : Outport  Port=4
  wires:
  Binary Logic1/1 -> Shifter3/1, Shifter2/1, Binary Logic3/2
  Constant/1 -> Shifter1/2
  Constant1/1 -> Shifter2/2
  Binary Logic2/1 -> Key_output3/1
  Binary Logic4/1 -> Binary Logic2/1
  key_input/1 -> Binary Logic3/1
  key_input1/1 -> Key_output/1, Binary Logic1/1
  z/1 -> Binary Logic5/1
  c/1 -> Binary Logic5/2
  key_input2/1 -> Key_output1/1
  key_input3/1 -> Shifter/1, Shifter1/1, Key_output2/1
  Binary Logic3/1 -> Binary Logic4/1
  Binary Logic5/1 -> Binary Logic2/2
  Constant2/1 -> Shifter/2
  Shifter1/1 -> Binary Logic6/1
  Shifter/1 -> Binary Logic6/2
  Binary Logic6/1 -> Binary Logic1/2
  Constant3/1 -> Shifter3/2
  Shifter2/1 -> Binary Logic7/1
  Shifter3/1 -> Binary Logic7/2
  Binary Logic7/1 -> Binary Logic4/2

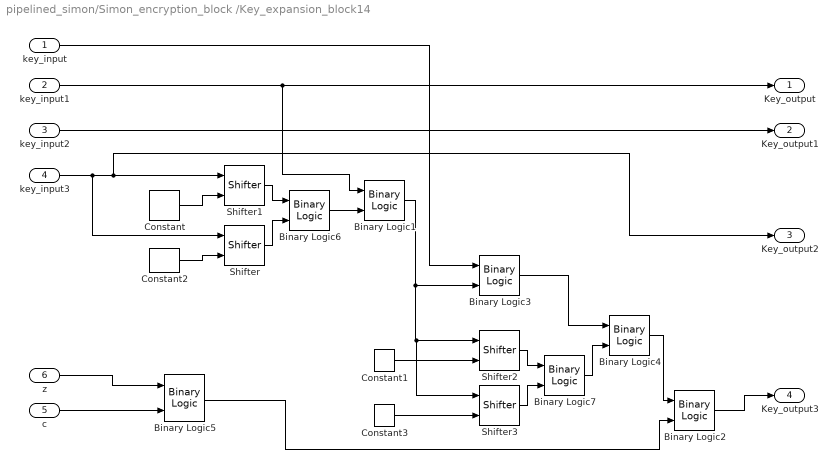
== system pipelined_simon/Simon_encryption_block /Key_expansion_block14 ==
  key_input : Inport
  key_input1 : Inport  Port=2
  key_input2 : Inport  Port=3
  key_input3 : Inport  Port=4
  c : Inport  Port=5
  z : Inport  Port=6
  Binary Logic{1..5} (5 alike) : shlslibv1/Math Functions/Binary Logic  syn_binlog_exp=a^b  synBlockType=primitive  synLatency=0  synBlockId=13
  Binary Logic6 : shlslibv1/Math Functions/Binary Logic  syn_binlog_exp=a|b  synBlockType=primitive  synLatency=0  synBlockId=13
  Binary Logic7 : shlslibv1/Math Functions/Binary Logic  syn_binlog_exp=a|b  synBlockType=primitive  synLatency=0  synBlockId=13
  Constant : shlslibv1/Sources/Constant  syn_cst_val=3  syn_cst_format=Specify  syn_cst_wl=4  syn_cst_fl=0  syn_cst_dt=unsigned  syn_cst_rnd=on  syn_cst_st=-1  synBlockType=primitive  synLatency=0  synBlockId=15
  Constant1 : shlslibv1/Sources/Constant  syn_cst_val=1  syn_cst_format=Specify  syn_cst_wl=4  syn_cst_fl=0  syn_cst_dt=unsigned  syn_cst_rnd=on  syn_cst_st=-1  synBlockType=primitive  synLatency=0  synBlockId=15
  Constant2 : shlslibv1/Sources/Constant  syn_cst_val=13  syn_cst_format=Specify  syn_cst_wl=4  syn_cst_fl=0  syn_cst_dt=unsigned  syn_cst_rnd=on  syn_cst_st=-1  synBlockType=primitive  synLatency=0  synBlockId=15
  Constant3 : shlslibv1/Sources/Constant  syn_cst_val=15  syn_cst_format=Specify  syn_cst_wl=4  syn_cst_fl=0  syn_cst_dt=unsigned  syn_cst_rnd=on  syn_cst_st=-1  synBlockType=primitive  synLatency=0  synBlockId=15
  Shifter : shlslibv1/Math Functions/Shifter  syn_shifter_opr=<<  syn_out_f=Automatic  syn_out_wl=16  syn_out_fl=8  syn_out_dt=signed  synBlockType=primitive  synLatency=0  synBlockId=12
  Shifter1 : shlslibv1/Math Functions/Shifter  syn_shifter_opr=>>  syn_out_f=Automatic  syn_out_wl=16  syn_out_fl=8  syn_out_dt=signed  synBlockType=primitive  synLatency=0  synBlockId=12
  Shifter2 : shlslibv1/Math Functions/Shifter  syn_shifter_opr=>>  syn_out_f=Automatic  syn_out_wl=16  syn_out_fl=8  syn_out_dt=signed  synBlockType=primitive  synLatency=0  synBlockId=12
  Shifter3 : shlslibv1/Math Functions/Shifter  syn_shifter_opr=<<  syn_out_f=Automatic  syn_out_wl=16  syn_out_fl=8  syn_out_dt=signed  synBlockType=primitive  synLatency=0  synBlockId=12
  Key_output : Outport
  Key_output1 : Outport  Port=2
  Key_output2 : Outport  Port=3
  Key_output3 : Outport  Port=4
  wires:
  Binary Logic1/1 -> Shifter3/1, Shifter2/1, Binary Logic3/2
  Constant/1 -> Shifter1/2
  Constant1/1 -> Shifter2/2
  Binary Logic2/1 -> Key_output3/1
  Binary Logic4/1 -> Binary Logic2/1
  key_input/1 -> Binary Logic3/1
  key_input1/1 -> Key_output/1, Binary Logic1/1
  z/1 -> Binary Logic5/1
  c/1 -> Binary Logic5/2
  key_input2/1 -> Key_output1/1
  key_input3/1 -> Shifter/1, Shifter1/1, Key_output2/1
  Binary Logic3/1 -> Binary Logic4/1
  Binary Logic5/1 -> Binary Logic2/2
  Constant2/1 -> Shifter/2
  Shifter1/1 -> Binary Logic6/1
  Shifter/1 -> Binary Logic6/2
  Binary Logic6/1 -> Binary Logic1/2
  Constant3/1 -> Shifter3/2
  Shifter2/1 -> Binary Logic7/1
  Shifter3/1 -> Binary Logic7/2
  Binary Logic7/1 -> Binary Logic4/2
